simulink model "Pokus11_Model_Input"  (Simulink 8.1)
settings: Solver=FixedStepDiscrete  StartTime=0.0  StopTime=10.0  FixedStep=1  RelTol=1e-3
undefined symbols (not defined in the file): External_Memory
settings Model: Creator=uzivatel  LastModifiedBy=uzivatel
settings DataIOCC: SignalLoggingSaveFormat=Dataset
settings OptimizationCC: ExpressionDepthLimit=128
settings DebuggingCC: FcnCallInpInsideContextMsg=EnableAllAsError
settings GRTTargetCC: CombineOutputUpdateFcns=on  GRTInterface=off

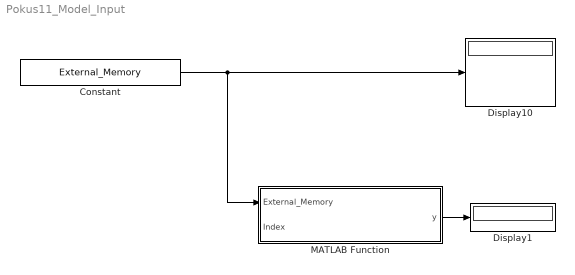
== system Pokus11_Model_Input ==
  Constant : Constant  Value=External_Memory
  Display1 : Display
  Display10 : Display
  MATLAB Function : MATLAB Function  TreatAsAtomicUnit=on
  wires:
  Constant/1 -> MATLAB Function/1(External_Memory), Display10/1
  MATLAB Function/1(y) -> Display1/1

== matlab function MATLAB Function ==
  data: y output double; External_Memory input double; Index input double
function y = fcn(External_Memory, Index)

    y = External_Memory(Index);

end
